simulink model "untitled"  (R2024b)
settings: Solver=VariableStepAuto  StartTime=0.0  StopTime=10.0  RelTol=1e-3
settings Model: Creator=DT User  LastModifiedBy=DT User

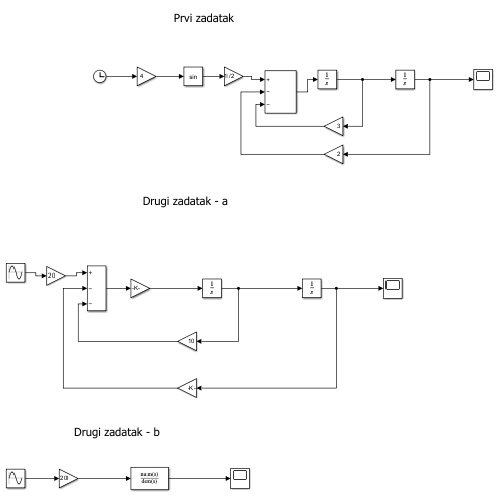
[thumbnail: Simulink's stored preview of the top-level diagram]
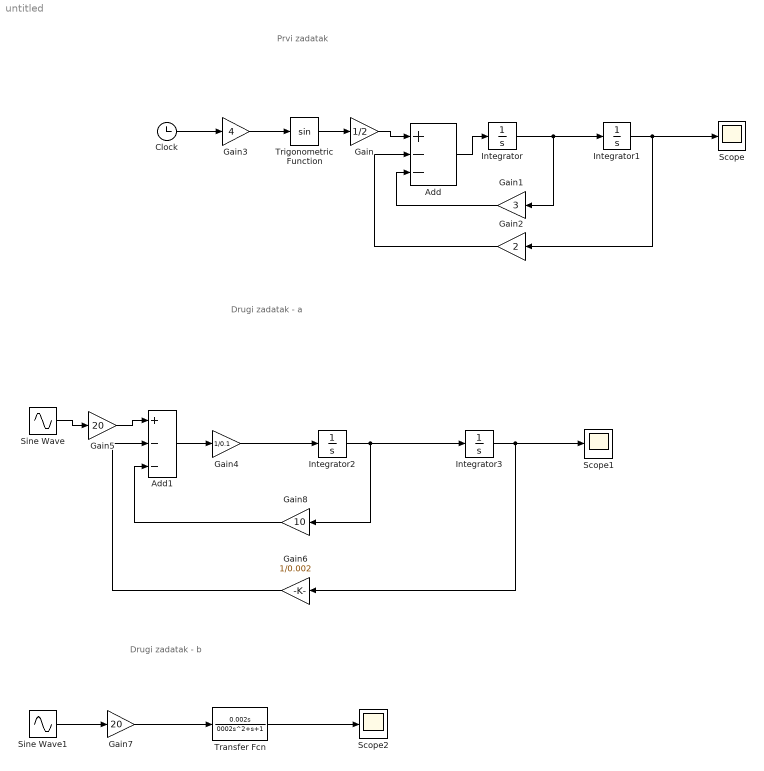
== system untitled ==
  note: Prvi zadatak
  note: Drugi zadatak - a
  note: Drugi zadatak - b
  Add : Sum  Inputs=+--
  Add1 : Sum  Inputs=+--
  Clock : Clock
  Gain : Gain  Gain=1/2
  Gain1 : Gain  Gain=3
  Gain2 : Gain  Gain=2
  Gain3 : Gain  Gain=4
  Gain4 : Gain  Gain=1/0.1
  Gain5 : Gain  Gain=20
  Gain6 : Gain  Gain=1/0.002
  Gain7 : Gain  Gain=20
  Gain8 : Gain  Gain=10
  Integrator : Integrator  InitialCondition=2
  Integrator1 : Integrator  InitialCondition=4
  Integrator2 : Integrator  InitialCondition=2
  Integrator3 : Integrator  InitialCondition=2
  Scope : Scope
  Scope1 : Scope
  Scope2 : Scope
  Sine Wave : Sin  SampleTime=0
  Sine Wave1 : Sin  SampleTime=0
  Transfer Fcn : TransferFcn  Numerator=[0.002 0]  Denominator=[0,0002 1 1]
  Trigonometric Function : Trigonometry
  wires:
  Integrator/1 -> Gain1/1, Integrator1/1
  Trigonometric Function/1 -> Gain/1
  Integrator1/1 -> Gain2/1, Scope/1
  Gain3/1 -> Trigonometric Function/1
  Clock/1 -> Gain3/1
  Gain/1 -> Add/1
  Gain1/1 -> Add/3
  Gain2/1 -> Add/2
  Add/1 -> Integrator/1
  Integrator2/1 -> Gain8/1, Integrator3/1
  Gain4/1 -> Integrator2/1
  Sine Wave/1 -> Gain5/1
  Add1/1 -> Gain4/1
  Gain5/1 -> Add1/1
  Integrator3/1 -> Scope1/1, Gain6/1
  Gain8/1 -> Add1/3
  Gain6/1 -> Add1/2
  Transfer Fcn/1 -> Scope2/1
  Gain7/1 -> Transfer Fcn/1
  Sine Wave1/1 -> Gain7/1
